simulink model "Glucose-Insulin Regulation Model"  (R2016b)
settings: Solver=ode1  StartTime=0.0  StopTime=5  FixedStep=.01  RelTol=1e-3  EnableMultiTasking=on
settings Model: Creator=My Account  LastModifiedBy=Swapnil
settings OptimizationCC: LifeSpan=inf
settings DebuggingCC: SFUnexpectedBacktrackingDiag=warning  SFNoUnconditionalDefaultTransitionDiag=warning  SFExecutionAtInitializationDiag=none
settings GRTTargetCC: TargetLangStandard=C89/C90 (ANSI)  GeneratePreprocessorConditionals=Disable all
settings ConfigComp: CovMetricSettings=dw  CovHtmlReporting=on  CovSaveCumulativeToWorkspaceVar=on  CovSaveSingleToWorkspaceVar=on  CovExternalEMLEnable=off

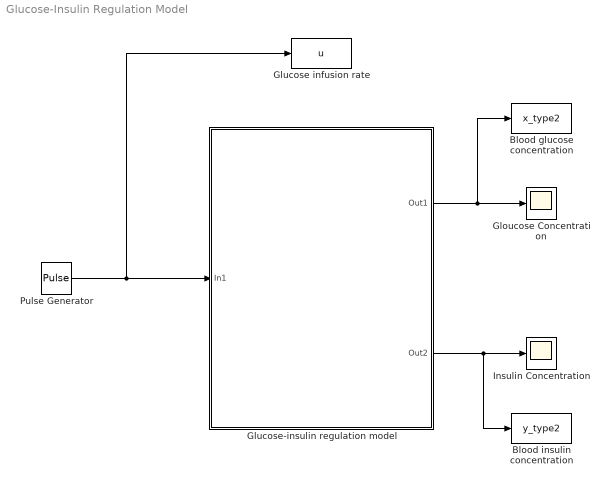
== system Glucose-Insulin Regulation Model ==
  "Blood glucose concentration " : ToWorkspace  VariableName=x_type2  SaveFormat=Timeseries  SampleTime=-1
  "Blood insulin concentration " : ToWorkspace  VariableName=y_type2  SaveFormat=Timeseries  SampleTime=-1
  Gloucose Concentration : Scope
  "Glucose infusion rate " : ToWorkspace  VariableName=u  SaveFormat=Timeseries  SampleTime=-1
  Glucose-insulin regulation model : Subsystem
  Insulin Concentration : Scope
  Pulse Generator : DiscretePulseGenerator  PulseType=Time based  Amplitude=100000  Period=5  PulseWidth=5  PhaseDelay=0.5
  wires:
  Pulse Generator/1 -> "Glucose infusion rate "/1, Glucose-insulin regulation model/1(In1)
  Glucose-insulin regulation model/1(Out1) -> "Blood glucose concentration "/1, Gloucose Concentration/1
  Glucose-insulin regulation model/2(Out2) -> "Blood insulin concentration "/1, Insulin Concentration/1

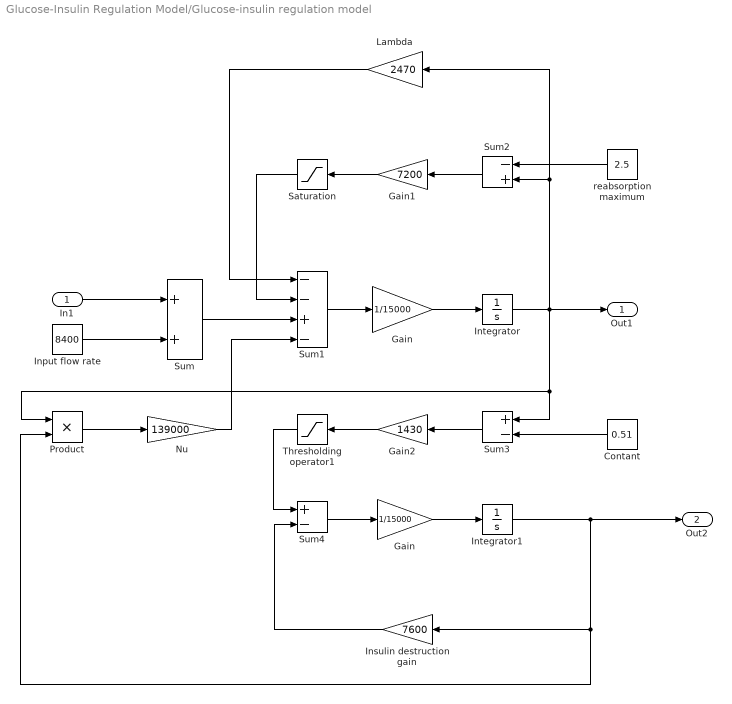
== system Glucose-Insulin Regulation Model/Glucose-insulin regulation model ==
  In1 : Inport
  Contant : Constant  Value=0.51
  Gain : Gain  Gain=1/15000
  "Gain " : Gain  Gain=1/15000
  Gain1 : Gain  Gain=7200
  Gain2 : Gain  Gain=1430
  Input flow rate : Constant  Value=8400
  Insulin destruction gain : Gain  Gain=7600
  Integrator : Integrator  InitialCondition=0.81
  Integrator1 : Integrator  InitialCondition=0.055
  Lambda : Gain  Gain=2470
  Nu : Gain  Gain=139000
  Product : Product
  Saturation : Saturate  UpperLimit=100000  LowerLimit=0
  Sum : Sum
  Sum1 : Sum  Inputs=--+-
  Sum2 : Sum  Inputs=-+
  Sum3 : Sum  Inputs=+-
  Sum4 : Sum  Inputs=+-
  Thresholding operator1 : Saturate  UpperLimit=100000  LowerLimit=0
  reabsorption maximum : Constant  Value=2.5
  Out1 : Outport
  Out2 : Outport  Port=2
  wires:
  In1/1 -> Sum/1
  Input flow rate/1 -> Sum/2
  Sum1/1 -> Gain/1
  Sum/1 -> Sum1/3
  Gain/1 -> Integrator/1
  Integrator/1 -> Sum3/1, Product/1, Sum2/2, Lambda/1, Out1/1
  Lambda/1 -> Sum1/1
  reabsorption maximum/1 -> Sum2/1
  Sum2/1 -> Gain1/1
  Gain1/1 -> Saturation/1
  Saturation/1 -> Sum1/2
  Contant/1 -> Sum3/2
  Sum3/1 -> Gain2/1
  Gain2/1 -> Thresholding operator1/1
  Thresholding operator1/1 -> Sum4/1
  Sum4/1 -> "Gain "/1
  "Gain "/1 -> Integrator1/1
  Integrator1/1 -> Insulin destruction gain/1, Product/2, Out2/1
  Insulin destruction gain/1 -> Sum4/2
  Product/1 -> Nu/1
  Nu/1 -> Sum1/4
